simulink model "andbot1dot2_voltage_loop"  (R2015b)
settings: Solver=VariableStepAuto  StartTime=0.0  StopTime=10  RelTol=1e-3
libraries: slctrlblks x1
settings Model: Creator=shangwei  LastModifiedBy=root

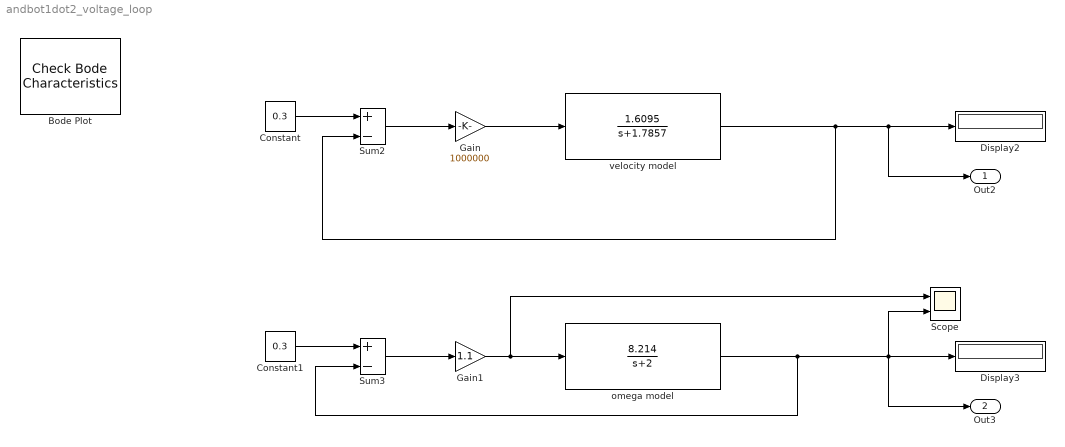
== system andbot1dot2_voltage_loop ==
  Bode Plot : slctrlblks/Model Verification/Check Bode  Characteristics  InstantiateOnLoad=on  SaveOperatingPoints=off  LinearizationIOs={'/velocity model', 1, 'out', 'on', '';'/Gain', 1, 'in', 'on', '';'/Gain1', 1, 'in', 'on', '';'/omega model', 1, 'out', 'on', ''}  LinearizeAt=SnapshotTimes  SnapshotTimes=[0]  TriggerType=rising  SampleTime=auto  RateConversionMethod=zoh  PreWarpFreq=10  UseExactDelayModel=off  UseFullBlockNameLabels=off  UseBusSignalLabels=off  enabled=on  stopWhenAssertionFail=off  export=off  ViewDlgPos=[464 -123 500 388]  OpenViewOnLoad=on  LaunchViewOnOpen=on  FrequencyUnits=rad/s  MagnitudeUnits=dB  PhaseUnits=deg  TimeUnits=seconds  EnableUpperBound=off  UpperBoundFrequencies=[]  UpperBoundMagnitudes=[]  EnableLowerBound=off  LowerBoundFrequencies=[]  LowerBoundMagnitudes=[]
  Constant : Constant  Value=0.3
  Constant1 : Constant  Value=0.3
  Display2 : Display
  Display3 : Display
  Gain : Gain  Gain=1000000
  Gain1 : Gain  Gain=1.1
  Scope : Scope  NumInputPorts=2
  Sum2 : Sum  Inputs=+-
  Sum3 : Sum  Inputs=+-
  omega model : TransferFcn  Numerator=[8.214]  Denominator=[1 2]
  velocity model : TransferFcn  Numerator=[1.6095]  Denominator=[1 1.7857]
  Out2 : Outport
  Out3 : Outport  Port=2
  wires:
  Sum2/1 -> Gain/1
  velocity model/1 -> Sum2/2, Display2/1, Out2/1
  Constant/1 -> Sum2/1
  Gain/1 -> velocity model/1
  Sum3/1 -> Gain1/1
  omega model/1 -> Sum3/2, Scope/2, Out3/1, Display3/1
  Constant1/1 -> Sum3/1
  Gain1/1 -> Scope/1, omega model/1
